simulink model "CruiseControl_TestSuite_Harness_Disengage_upon_braking"  (R2019b)
settings: Solver=FixedStepDiscrete  StartTime=0.0  StopTime=10  FixedStep=0.1  RelTol=1e-3  EnableMultiTasking=on
settings Model: Creator=patcanny  LastModifiedBy=patcanny
settings DataIOCC: LimitDataPoints=on  SaveFormat=Array  SaveOutput=off  SaveTime=off  ReturnWorkspaceOutputs=off
settings OptimizationCC: DefaultParameterBehavior=Inlined  InlineInvariantSignals=on  ExpressionDepthLimit=2147483647  InitFltsAndDblsToZero=on  NoFixptDivByZeroProtection=on  LifeSpan=inf  EfficientTunableParamExpr=on
settings DebuggingCC: SignalInfNanChecking=warning  SaveWithParameterizedLinksMsg=none  UnderspecifiedInitializationDetection=Classic  MergeDetectMultiDrivingBlocksExec=none  SolverPrmCheckMsg=warning  FcnCallInpInsideContextMsg=warning  UniqueDataStoreMsg=warning  AllowSymbolicDim=off  StateNameClashWarn=warning  StrictBusMsg=ErrorOnBusTreatedAsVector  SFUnexpectedBacktrackingDiag=warning  SFNoUnconditionalDefaultTransitionDiag=warning  SFExecutionAtInitializationDiag=none  ArithmeticOperatorsInVariantConditions=warning
settings HardwareCC: ProdBitPerPointer=32  ProdBitPerSizeT=32  ProdBitPerPtrDiffT=32  ProdLargestAtomicFloat=None  ProdIntDivRoundTo=Undefined  ProdEndianess=Unspecified  ProdWordSize=32  ProdHWDeviceType=32-bit Generic
settings ModelReferenceCC: ModelReferenceNumInstancesAllowed=Single  PropagateSignalLabelsOutOfModel=off
settings SFSimCC: SimUseLocalCustomCode=off  SimParseCustomCode=off  MATLABDynamicMemAlloc=off  CustomCodeUndefinedFunction=UseInterfaceOnly
settings RTWCC: SystemTargetFile=ert.tlc  TemplateMakefile=ert_default_tmf  GenerateReport=on  RTWUseLocalCustomCode=off  IncludeHyperlinkInReport=on  LaunchReport=on  PortableWordSizes=on  GenerateTraceInfo=on  GenerateTraceReport=on  GenerateTraceReportSl=on  GenerateTraceReportSf=on  GenerateTraceReportEml=on
settings CodeAppCC: IgnoreCustomStorageClasses=off  CustomSymbolStrGlobalVar=$N$M  StateflowObjectComments=on
settings ERTTargetCC: MultiwordLength=2048  GenerateSampleERTMain=on  InlinedParameterPlacement=NonHierarchical  ERTCustomFileTemplate=example_file_process.tlc  ConvertIfToSwitch=off  SuppressUnreachableDefaultCases=off
settings ConfigComp: CovScope=ReferencedModels  CovIncludeTopModel=off  CovMetricSettings=dcme  CovEnableCumulative=off  CovExternalEMLEnable=off  CovSFcnEnable=off  DVMode=DesignErrorDetection  DVMaxProcessTime=3000  DVDisplayUnsatisfiableObjectives=on  DVAutomaticStubbing=off  DVMakeOutputFilesUnique=off  DVModelCoverageObjectives=MCDC  DVMaxTestCaseSteps=500  DVTestSuiteOptimization=CombinedObjectives  DVAssertions=EnableAll  DVProofAssumptions=EnableAll  DVIgnoreCovSatisfied=on  DVCoverageDataFile=CruiseControlCovManual.cvt  DVDetectDeadLogic=on  DVDetectActiveLogic=on  DVDetectIntegerOverflow=off  DVMaxViolationSteps=50  DVSaveExpectedOutput=on  DVHarnessModelFileName=$ModelName$_harness_SLDV  DVReportIncludeGraphics=on  DVRebuildModelRepresentation=Always

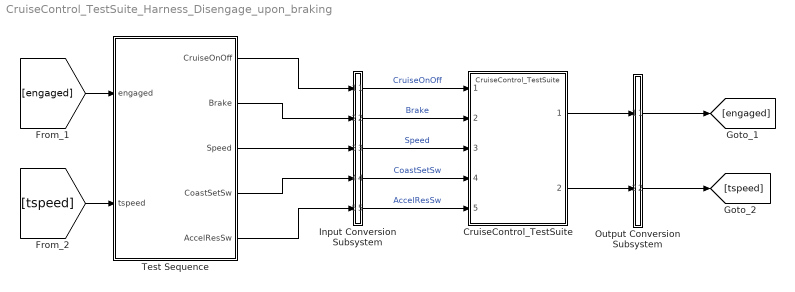
== system CruiseControl_TestSuite_Harness_Disengage_upon_braking ==
  CruiseControl_TestSuite : ModelReference  ModelNameDialog=CruiseControl_TestSuite  SimulationMode=Normal  ModelReferenceVersion=1.481
  Input Conversion Subsystem : Subsystem  Tag=__SLT_ICS__  Description=|
      | Signal spec.
      | and routing
      settings: AttributesFormatString=%<Description>
  Output Conversion Subsystem : Subsystem  Tag=__SLT_OCS__  Description=|
      | Signal spec.
      | and routing
      settings: AttributesFormatString=%<Description>
  Test Sequence : Test Sequence  TreatAsAtomicUnit=on
  wires:
  [engaged] -> Test Sequence/1(engaged)
  Output Conversion Subsystem/1(Outport_1) -> [engaged]
  Output Conversion Subsystem/2(Outport_2) -> [tspeed]
  Input Conversion Subsystem/1(Outport_1) -> CruiseControl_TestSuite/1  "CruiseOnOff"
  Input Conversion Subsystem/2(Outport_2) -> CruiseControl_TestSuite/2  "Brake"
  Input Conversion Subsystem/3(Outport_3) -> CruiseControl_TestSuite/3  "Speed"
  Input Conversion Subsystem/4(Outport_4) -> CruiseControl_TestSuite/4  "CoastSetSw"
  Input Conversion Subsystem/5(Outport_5) -> CruiseControl_TestSuite/5  "AccelResSw"
  CruiseControl_TestSuite/1 -> Output Conversion Subsystem/1(Inport_1)
  CruiseControl_TestSuite/2 -> Output Conversion Subsystem/2(Inport_2)
  [tspeed] -> Test Sequence/2(tspeed)
  Test Sequence/3(Speed) -> Input Conversion Subsystem/3(Inport_3)
  Test Sequence/2(Brake) -> Input Conversion Subsystem/2(Inport_2)
  Test Sequence/4(CoastSetSw) -> Input Conversion Subsystem/4(Inport_4)
  Test Sequence/1(CruiseOnOff) -> Input Conversion Subsystem/1(Inport_1)
  Test Sequence/5(AccelResSw) -> Input Conversion Subsystem/5(Inport_5)

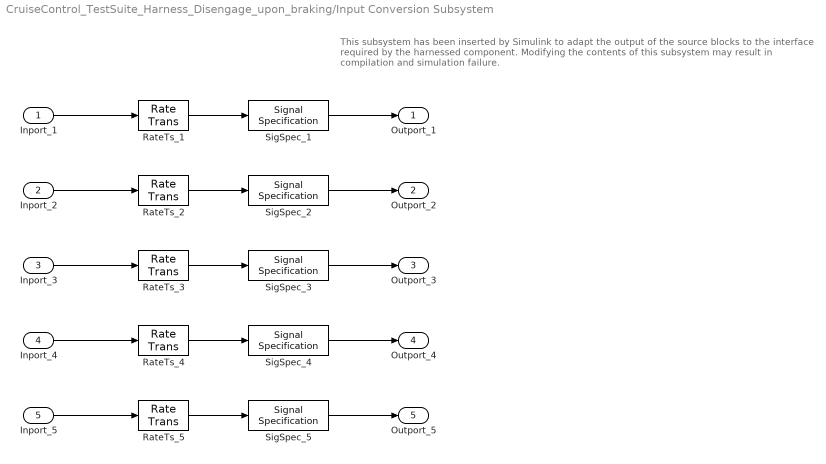
== system CruiseControl_TestSuite_Harness_Disengage_upon_braking/Input Conversion Subsystem ==
  note: This subsystem has been inserted by Simulink to adapt the output of the source blocks to the interface required by the harnessed component.
      |  Modifying the contents of this subsystem may result in compilation and simulation failure.
  Inport_1 : Inport
  Inport_2 : Inport  Port=2
  Inport_3 : Inport  Port=3
  Inport_4 : Inport  Port=4
  Inport_5 : Inport  Port=5
  RateTs_{1..5} (5 alike) : RateTransition  OutPortSampleTime=0.1
  SigSpec_{1..2,4..5} (4 alike) : SignalSpecification  OutDataTypeStr=boolean  Dimensions=[1]  SampleTime=0.1
  SigSpec_3 : SignalSpecification  OutDataTypeStr=uint8  Dimensions=[1]  SampleTime=0.1
  Outport_1 : Outport
  Outport_2 : Outport  Port=2
  Outport_3 : Outport  Port=3
  Outport_4 : Outport  Port=4
  Outport_5 : Outport  Port=5
  wires:
  SigSpec_1/1 -> Outport_1/1
  RateTs_1/1 -> SigSpec_1/1
  Inport_1/1 -> RateTs_1/1
  SigSpec_2/1 -> Outport_2/1
  RateTs_2/1 -> SigSpec_2/1
  Inport_2/1 -> RateTs_2/1
  SigSpec_3/1 -> Outport_3/1
  RateTs_3/1 -> SigSpec_3/1
  Inport_3/1 -> RateTs_3/1
  SigSpec_4/1 -> Outport_4/1
  RateTs_4/1 -> SigSpec_4/1
  Inport_4/1 -> RateTs_4/1
  SigSpec_5/1 -> Outport_5/1
  RateTs_5/1 -> SigSpec_5/1
  Inport_5/1 -> RateTs_5/1

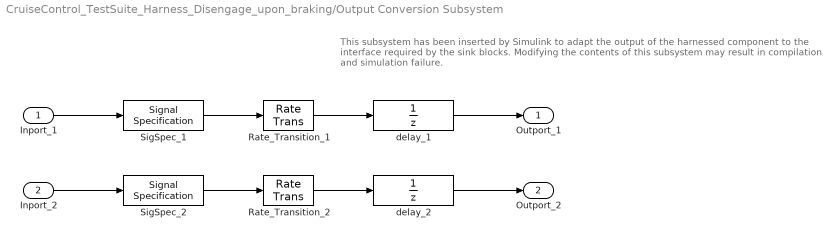
== system CruiseControl_TestSuite_Harness_Disengage_upon_braking/Output Conversion Subsystem ==
  note: This subsystem has been inserted by Simulink to adapt the output of the harnessed component to the interface required by the sink blocks.
      |  Modifying the contents of this subsystem may result in compilation and simulation failure.
  Inport_1 : Inport
  Inport_2 : Inport  Port=2
  Rate_Transition_1 : RateTransition  OutPortSampleTimeOpt=Inherit
  Rate_Transition_2 : RateTransition  OutPortSampleTimeOpt=Inherit
  SigSpec_1 : SignalSpecification  OutDataTypeStr=boolean  Dimensions=[1]  SampleTime=0.1
  SigSpec_2 : SignalSpecification  OutDataTypeStr=uint8  Dimensions=[1]  SampleTime=0.1
  delay_1 : UnitDelay  SampleTime=-1
  delay_2 : UnitDelay  SampleTime=-1
  Outport_1 : Outport
  Outport_2 : Outport  Port=2
  wires:
  Inport_1/1 -> SigSpec_1/1
  SigSpec_1/1 -> Rate_Transition_1/1
  Rate_Transition_1/1 -> delay_1/1
  delay_1/1 -> Outport_1/1
  Inport_2/1 -> SigSpec_2/1
  SigSpec_2/1 -> Rate_Transition_2/1
  Rate_Transition_2/1 -> delay_2/1
  delay_2/1 -> Outport_2/1

== stateflow chart CruiseControl_TestSuite_Harness_Disengage_upon_braking/Test Sequence ==
  settings: updateMethod=DISCRETE  sampleTime=0.1  stateMachineType=SIMPLIFIED_MACHINE
  state Run
    %% Initialize data outputs.
    CruiseOnOff = false;
    Brake = false;
    Speed = uint8(0);
    CoastSetSw = false;
    AccelResSw = false;
  state step_1
    % Enable cruise control
    CruiseOnOff = true;
    Speed = uint8(50);
  state step_2
    % Verify not engaged yet
    verify(~engaged)
  state step_3
    CoastSetSw = true;
  state step_4
    verify(engaged)
  state step_5
    Brake = true;
  state step_6
    verify(~engaged)
  (default) -> Run
  Run -> step_1 : [
      | after(1,sec)
      | ]
  step_1 -> step_2 : [
      | after(1,sec)
      | ]
  step_2 -> step_3
  step_3 -> step_4 : [
      | after(1,sec)
      | ]
  step_4 -> step_5
  step_5 -> step_6 : [
      | after(0.2,sec)
      | ]
  data: engaged input boolean size=[1]; tspeed input uint8 size=[1]; CruiseOnOff output boolean size=[1]; Brake output boolean size=[1]; Speed output uint8 size=[1]; CoastSetSw output boolean size=[1]; AccelResSw output boolean size=[1]
